simulink model "test8_sub_named_with_slash_diff"  (R2016b)
settings: Solver=VariableStepAuto  StartTime=0.0  StopTime=10.0  RelTol=1e-3
settings Model: Creator=gm  LastModifiedBy=gm

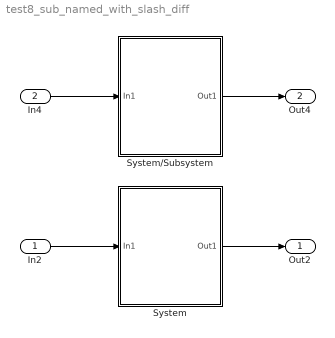
== system test8_sub_named_with_slash_diff ==
  In2 : Inport
  In4 : Inport  Port=2
  System : Subsystem
  System/Subsystem : Subsystem
  Out2 : Outport
  Out4 : Outport  Port=2
  wires:
  In2/1 -> System/1(In1)
  System/1(Out1) -> Out2/1
  System/Subsystem/1(Out1) -> Out4/1
  In4/1 -> System/Subsystem/1(In1)

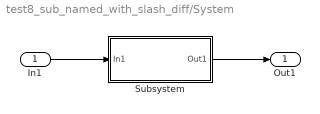
== system test8_sub_named_with_slash_diff/System ==
  In1 : Inport
  Subsystem : Subsystem
  Out1 : Outport
  wires:
  In1/1 -> Subsystem/1(In1)
  Subsystem/1(Out1) -> Out1/1

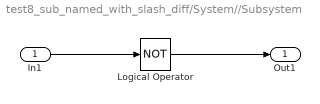
== system test8_sub_named_with_slash_diff/System//Subsystem ==
  In1 : Inport
  Logical Operator : Logic  Operator=NOT  AllPortsSameDT=off  OutDataTypeStr=boolean
  Out1 : Outport
  wires:
  In1/1 -> Logical Operator/1
  Logical Operator/1 -> Out1/1

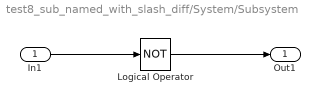
== system test8_sub_named_with_slash_diff/System/Subsystem ==
  In1 : Inport
  Logical Operator : Logic  Operator=NOT  AllPortsSameDT=off  OutDataTypeStr=boolean
  Out1 : Outport
  wires:
  In1/1 -> Logical Operator/1
  Logical Operator/1 -> Out1/1
